simulink model "sampleModel1584"  (R2023a)
settings: Solver=VariableStepAuto  StartTime=0.0  StopTime=10.0  RelTol=1e-3
libraries: hdlsllib x6, simulink x1
settings Model: Creator=user1  LastModifiedBy=user1

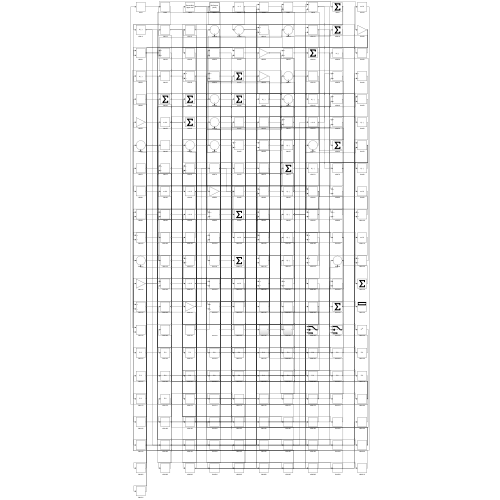
[thumbnail: Simulink's stored preview of the top-level diagram]
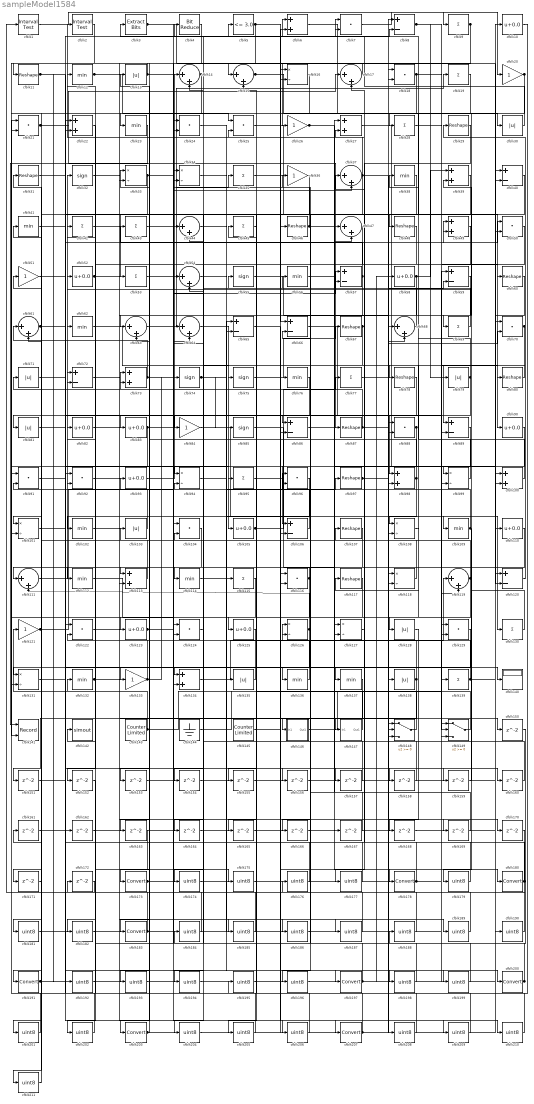
== system sampleModel1584 ==
  cfblk1 : hdlsllib/Logic and Bit Operations/Interval Test  IntervalClosedRight=on  uplimit=0.5  IntervalClosedLeft=on  lowlimit=-0.5  OutDataTypeStr=boolean
  cfblk{10,52,58,82..83,90,93,105,110,123,125} (11 alike) : Bias  Bias=0.0  SaturateOnIntegerOverflow=off
  cfblk{6,22,27,39,49,73,98,100,113,134} (10 alike) : Sum
  cfblk{16,33..34,94,99,101,108,118,126..127,131} (11 alike) : Product  Inputs=*/  RndMeth=Zero  SaturateOnIntegerOverflow=on
  cfblk{12,23,38,41,56,62,76,102,109,112,114,132,136..137} (14 alike) : MinMax
  cfblk{13,30,71,79,81,103,128,135,138} (9 alike) : Abs  SaturateOnIntegerOverflow=off
  cfblk{7,18,21,24..25,50,70,88,91..92,96,104,116,122,124,129} (16 alike) : DotProduct  OutDataTypeStr=Inherit: Inherit via internal rule
  cfblk{8,40,57,59,65..66,72,86,89,106,120} (11 alike) : Sum  Inputs=+-
  cfblk{11,29,31,46,48,60,67,78,80,87,97,107,117} (13 alike) : Reshape
  cfblk{14..15,17,37,44,47,54,61,63..64,68,111,119} (13 alike) : Sum  Inputs=|++
  cfblk{9,19,28,35,42..43,45,53,69,77,95,115,130,139} (14 alike) : Sum  Inputs=+
  cfblk{20,26,36,51,84,121,133} (7 alike) : Gain
  cfblk140 : Display
  cfblk141 : Record  FileSettingsInternal="{\"entries\":[{\"content\":{\"excelSettings\":{\"content\":{},\"type\":\"Streamout.ExcelSettings\"}},\"type\":\"Streamout.FileSettingStorage\",\"uuid\":\"\"}],\"packageUris\":[\"http:\\/\\/schema.mathworks.com\\/mf0\\/streamout_blocks\\/R2020a\"],\"version\":\"1.0\"}"  Layout=[1 1]  SignalsInternal="{\"entries\":[{\"content\":{\"signals\":[{\"content\":{\"blockPath\":[],\"dimensions\":[1],\"domain\":\"\",\"lineColor\":\"#a2142f\",\"plots\":[1],\"port\":1,\"signalID\":2030,\"signalName\":\"XY Graph:1\"},\"type\":\"RecordBlkView.Signal\",\"uuid\":\"\"},{\"content\":{\"blockPath\":[],\"dimensions\":[1],\"domain\":\"\",\"lineColor\":\"#139fff\",\"plots\":[1],\"port\":2,\"signalID\":2033,\"signalName\":\"XY Graph:2\"},\"type\":\"RecordBlkView.Signal\",\"uuid\":\"\"}]},\"type\":\"RecordBlkView.InputSignals\",\"uuid\":\"\"}],\"packageUris\":[\"http:\\/\\/schema.mathworks.com\\/mf0\\/streamout_blocks\\/R2020a\"],\"version\":\"1.0\"}"  VisualizationBindings="{\"xyplotplugin\":{\"info\":[{\"series\":[{\"bindingParametersList\":[{\"parameter\":\"X-Axis\",\"signalID\":2030,\"signalName\":\"XY Graph:1\"},{\"parameter\":\"Y-Axis\",\"signalID\":2033,\"signalName\":\"XY Graph:2\"}],\"seriesID\":50669}],\"subplotID\":1}]}}"  CompatibilityTag=XY  st=-1
  cfblk142 : ToWorkspace  VariableName=simout  SaveFormat=Timeseries  SampleTime=-1
  cfblk143 : hdlsllib/Sources/Counter Limited  uplimit=7  tsamp=-1
  cfblk144 : Ground
  cfblk145 : hdlsllib/Sources/Counter Limited  uplimit=7  tsamp=-1
  cfblk146 : Subsystem
      settings: LibrarySourceBlock=|
      | hdlsllib/Ports &
      | Subsystems/Subsystem
  cfblk147 : Subsystem
      settings: LibrarySourceBlock=|
      | hdlsllib/Ports &
      | Subsystems/Subsystem
  cfblk148 : Switch  SaturateOnIntegerOverflow=off  InputSameDT=off
  cfblk149 : Switch  SaturateOnIntegerOverflow=off  InputSameDT=off
  cfblk{150..172} (23 alike) : Delay  SampleTime=1
  cfblk{173,178,180,183,191,197,200,203,207} (9 alike) : DataTypeConversion  SaturateOnIntegerOverflow=off  RndMeth=Floor
  cfblk{174..177,179,181..182,184..190,192..196,198..199,201..202,204..206,208..211} (30 alike) : DataTypeConversion  OutDataTypeStr=uint8  SaturateOnIntegerOverflow=off  RndMeth=Floor
  cfblk2 : hdlsllib/Logic and Bit Operations/Interval Test  IntervalClosedRight=on  uplimit=0.5  IntervalClosedLeft=on  lowlimit=-0.5  OutDataTypeStr=boolean
  cfblk3 : simulink/Logic and Bit Operations/Extract Bits  bitsToExtract=Upper half  numBits=8  bitIdxRange=[0 7]  outScalingMode=Preserve fixed-point scaling
      settings: LibrarySourceBlock=|
      | hdlsllib/Logic and Bit
      | Operations/Extract Bits
  cfblk{32,55,74..75,85} (5 alike) : Signum
  cfblk4 : hdlsllib/Logic and Bit Operations/Bit Reduce  mode=AND
  cfblk5 : hdlsllib/Logic and Bit Operations/Compare To Constant  relop=<=  const=3.0  OutDataTypeStr=boolean
  wires:
  cfblk92/1 -> cfblk207/1
  cfblk27/1 -> cfblk99/1
  cfblk12/1 -> cfblk25/1, cfblk88/2
  cfblk103/1 -> cfblk32/1
  cfblk100/1 -> cfblk3/1
  cfblk115/1 -> cfblk173/1
  cfblk25/1 -> cfblk87/1
  cfblk78/1 -> cfblk81/1
  cfblk34/1 -> cfblk197/1
  cfblk111/1 -> cfblk62/1
  cfblk66/1 -> cfblk98/1
  cfblk64/1 -> cfblk105/1
  cfblk118/1 -> cfblk61/1
  cfblk35/1 -> cfblk90/1
  cfblk99/1 -> cfblk38/1
  cfblk75/1 -> cfblk67/1
  cfblk119/1 -> cfblk126/1, cfblk94/2, cfblk193/1
  cfblk98/1 -> cfblk108/1, cfblk73/2
  cfblk59/1 -> cfblk123/1
  cfblk108/1 -> cfblk117/1
  cfblk43/1 -> cfblk35/1
  cfblk120/1 -> cfblk29/1
  cfblk65/1 -> cfblk180/1
  cfblk93/1 -> cfblk14/1
  cfblk1/1 -> cfblk20/1
  cfblk147/1(Out1) -> cfblk55/1
  cfblk62/1 -> cfblk75/1
  cfblk39/1 -> cfblk125/1
  cfblk23/1 -> cfblk141/1
  cfblk56/1 -> cfblk178/1
  cfblk91/1 -> cfblk200/1
  cfblk63/1 -> cfblk19/1
  cfblk26/1 -> cfblk158/1, cfblk159/1
  cfblk84/1 -> cfblk130/1
  cfblk19/1 -> cfblk101/1
  cfblk105/1 -> cfblk77/1, cfblk209/1
  cfblk49/1 -> cfblk146/1(In1)
  cfblk5/1 -> cfblk66/1, cfblk124/2
  cfblk31/1 -> cfblk84/1
  cfblk30/1 -> cfblk5/1
  cfblk134/1 -> cfblk119/1
  cfblk124/1 -> cfblk24/1
  cfblk6/1 -> cfblk30/1
  cfblk143/1 -> cfblk121/1, cfblk106/2
  cfblk58/1 -> cfblk137/1, cfblk39/1
  cfblk121/1 -> cfblk44/1, cfblk50/1
  cfblk61/1 -> cfblk6/1, cfblk95/1
  cfblk70/1 -> cfblk94/1, cfblk89/1, cfblk128/1
  cfblk20/1 -> cfblk48/1, cfblk69/1, cfblk22/2
  cfblk18/1 -> cfblk149/1, cfblk153/1
  cfblk22/1 -> cfblk112/1
  cfblk144/1 -> cfblk98/2
  cfblk107/1 -> cfblk134/1
  cfblk87/1 -> cfblk71/1, cfblk15/2, cfblk59/2
  cfblk50/1 -> cfblk102/1
  cfblk88/1 -> cfblk113/1, cfblk164/1
  cfblk95/1 -> cfblk127/1
  cfblk138/1 -> cfblk44/2, cfblk165/1, cfblk166/1
  cfblk73/1 -> cfblk31/1, cfblk37/2
  cfblk21/1 -> cfblk47/1, cfblk17/1
  cfblk126/1 -> cfblk111/2, cfblk154/1
  cfblk110/1 -> cfblk136/1
  cfblk60/1 -> cfblk120/2
  cfblk13/1 -> cfblk11/1, cfblk86/1
  cfblk89/1 -> cfblk106/1
  cfblk14/1 -> cfblk23/1, cfblk21/2
  cfblk80/1 -> cfblk78/1
  cfblk104/1 -> cfblk183/1
  cfblk3/1 -> cfblk110/1, cfblk8/2
  cfblk46/1 -> cfblk24/2, cfblk100/2
  cfblk74/1 -> cfblk85/1, cfblk170/1
  cfblk117/1 -> cfblk141/2
  cfblk7/1 -> cfblk9/1
  cfblk116/1 -> cfblk111/1, cfblk181/1
  cfblk16/1 -> cfblk191/1
  cfblk68/1 -> cfblk4/1
  cfblk136/1 -> cfblk72/1
  cfblk132/1 -> cfblk72/2, cfblk147/1(In1)
  cfblk2/1 -> cfblk101/2
  cfblk28/1 -> cfblk80/1
  cfblk145/1 -> cfblk49/1
  cfblk38/1 -> cfblk53/1
  cfblk123/1 -> cfblk7/1, cfblk198/1
  cfblk52/1 -> cfblk148/3, cfblk185/1
  cfblk94/1 -> cfblk135/1
  cfblk67/1 -> cfblk127/2, cfblk17/2, cfblk155/1
  cfblk85/1 -> cfblk139/1
  cfblk36/1 -> cfblk63/1
  cfblk135/1 -> cfblk131/1
  cfblk101/1 -> cfblk140/1
  cfblk9/1 -> cfblk26/1, cfblk33/2
  cfblk97/1 -> cfblk118/1, cfblk109/1, cfblk70/2
  cfblk24/1 -> cfblk108/2
  cfblk37/1 -> cfblk2/1, cfblk89/2, cfblk196/1
  cfblk55/1 -> cfblk68/2
  cfblk130/1 -> cfblk52/1
  cfblk114/1 -> cfblk97/1
  cfblk148/1 -> cfblk107/1
  cfblk83/1 -> cfblk57/2, cfblk163/1, cfblk206/1, cfblk211/1
  cfblk69/1 -> cfblk36/1
  cfblk15/1 -> cfblk28/1, cfblk7/2
  cfblk127/1 -> cfblk37/1
  cfblk79/1 -> cfblk57/1, cfblk171/1
  cfblk112/1 -> cfblk134/2
  cfblk4/1 -> cfblk83/1
  cfblk17/1 -> cfblk15/1
  cfblk48/1 -> cfblk114/1
  cfblk149/1 -> cfblk96/1
  cfblk90/1 -> cfblk131/2
  cfblk44/1 -> cfblk149/2
  cfblk146/1(Out1) -> cfblk59/1
  cfblk106/1 -> cfblk41/1
  cfblk53/1 -> cfblk64/2
  cfblk133/1 -> cfblk12/1, cfblk74/1
  cfblk113/1 -> cfblk82/1
  cfblk76/1 -> cfblk203/1
  cfblk139/1 -> cfblk10/1, cfblk33/1
  cfblk33/1 -> cfblk88/1, cfblk201/1
  cfblk11/1 -> cfblk50/2, cfblk192/1
  cfblk47/1 -> cfblk133/1
  cfblk71/1 -> cfblk49/2
  cfblk57/1 -> cfblk43/1, cfblk113/2
  cfblk109/1 -> cfblk73/1, cfblk179/1
  cfblk8/1 -> cfblk60/1, cfblk79/1
  cfblk72/1 -> cfblk150/1
  cfblk137/1 -> cfblk151/1
  cfblk96/1 -> cfblk152/1
  cfblk153/1 -> cfblk100/1
  cfblk154/1 -> cfblk47/2
  cfblk155/1 -> cfblk25/2
  cfblk41/1 -> cfblk156/1
  cfblk156/1 -> cfblk119/2
  cfblk81/1 -> cfblk157/1
  cfblk157/1 -> cfblk126/2
  cfblk158/1 -> cfblk64/1
  cfblk159/1 -> cfblk39/2
  cfblk32/1 -> cfblk160/1
  cfblk160/1 -> cfblk14/2
  cfblk161/1 -> cfblk68/1
  cfblk131/1 -> cfblk162/1
  cfblk162/1 -> cfblk6/2
  cfblk164/1 -> cfblk118/2
  cfblk165/1 -> cfblk148/2
  cfblk166/1 -> cfblk129/2
  cfblk86/1 -> cfblk167/1
  cfblk167/1 -> cfblk66/2
  cfblk128/1 -> cfblk168/1
  cfblk168/1 -> cfblk120/1
  cfblk102/1 -> cfblk169/1
  cfblk169/1 -> cfblk27/1
  cfblk171/1 -> cfblk61/2
  cfblk172/1 -> cfblk1/1
  cfblk173/1 -> cfblk99/2, cfblk46/1
  cfblk129/1 -> cfblk174/1
  cfblk174/1 -> cfblk115/1
  cfblk122/1 -> cfblk175/1
  cfblk175/1 -> cfblk116/2
  cfblk170/1 -> cfblk176/1
  cfblk176/1 -> cfblk122/1
  cfblk29/1 -> cfblk177/1
  cfblk177/1 -> cfblk122/2
  cfblk178/1 -> cfblk22/1, cfblk116/1
  cfblk179/1 -> cfblk56/1
  cfblk180/1 -> cfblk142/1, cfblk27/2, cfblk124/1
  cfblk181/1 -> cfblk65/1
  cfblk152/1 -> cfblk182/1
  cfblk182/1 -> cfblk65/2
  cfblk183/1 -> cfblk172/1, cfblk8/1, cfblk129/1
  cfblk150/1 -> cfblk184/1
  cfblk184/1 -> cfblk104/1
  cfblk185/1 -> cfblk104/2
  cfblk54/1 -> cfblk186/1
  cfblk186/1 -> cfblk18/2
  cfblk82/1 -> cfblk187/1
  cfblk187/1 -> cfblk54/1
  cfblk188/1 -> cfblk54/2
  cfblk42/1 -> cfblk189/1
  cfblk189/1 -> cfblk18/1
  cfblk190/1 -> cfblk42/1
  cfblk191/1 -> cfblk86/2, cfblk138/1
  cfblk192/1 -> cfblk16/1
  cfblk193/1 -> cfblk16/2
  cfblk40/1 -> cfblk194/1
  cfblk194/1 -> cfblk149/3
  cfblk10/1 -> cfblk195/1
  cfblk195/1 -> cfblk40/1
  cfblk196/1 -> cfblk40/2
  cfblk197/1 -> cfblk13/1, cfblk58/1
  cfblk198/1 -> cfblk34/1
  cfblk151/1 -> cfblk199/1
  cfblk199/1 -> cfblk34/2
  cfblk200/1 -> cfblk188/1, cfblk96/2, cfblk132/1
  cfblk201/1 -> cfblk91/1
  cfblk163/1 -> cfblk202/1
  cfblk202/1 -> cfblk91/2
  cfblk203/1 -> cfblk190/1, cfblk70/1, cfblk148/1, cfblk63/2
  cfblk125/1 -> cfblk204/1
  cfblk204/1 -> cfblk76/1
  cfblk45/1 -> cfblk205/1
  cfblk205/1 -> cfblk103/1
  cfblk206/1 -> cfblk45/1
  cfblk207/1 -> cfblk21/1, cfblk93/1
  cfblk77/1 -> cfblk208/1
  cfblk208/1 -> cfblk92/1
  cfblk209/1 -> cfblk92/2
  cfblk51/1 -> cfblk210/1
  cfblk210/1 -> cfblk161/1
  cfblk211/1 -> cfblk51/1

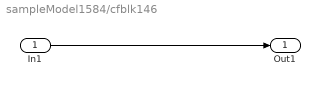
== system sampleModel1584/cfblk146 ==
  In1 : Inport
  Out1 : Outport
  wires:
  In1/1 -> Out1/1

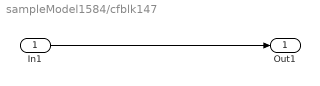
== system sampleModel1584/cfblk147 ==
  In1 : Inport
  Out1 : Outport
  wires:
  In1/1 -> Out1/1
